simulink model "GIM81115_6_motor_model"  (R2024b)
settings: Solver=VariableStepAuto  StartTime=0.0  StopTime=10.0  RelTol=1e-3
libraries: aru_toolbox x1
settings Model: Creator=claro  LastModifiedBy=claro

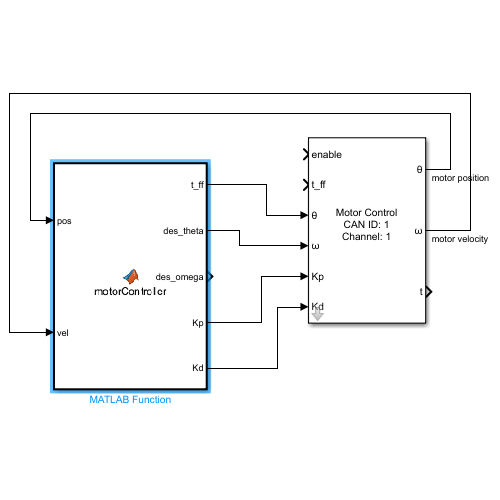
[thumbnail: Simulink's stored preview of the top-level diagram]
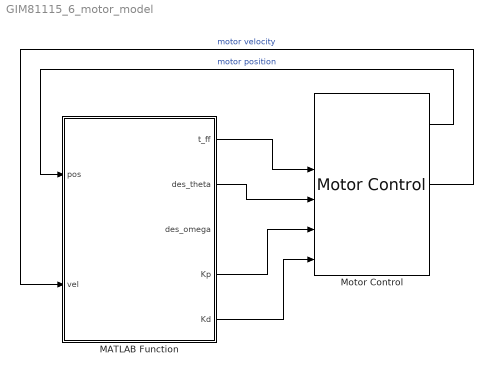
== system GIM81115_6_motor_model ==
  MATLAB Function : MATLAB Function  TreatAsAtomicUnit=on
  Motor Control : aru_toolbox/Motor Control  id=1  channel=1  offset=0
      settings: SourceProductName=ARU Toolbox
  wires:
  Motor Control/2 -> MATLAB Function/2(vel)  "motor velocity"
  Motor Control/1 -> MATLAB Function/1(pos)  "motor position"
  MATLAB Function/4(Kp) -> Motor Control/5
  MATLAB Function/5(Kd) -> Motor Control/6
  MATLAB Function/2(des_theta) -> Motor Control/4
  MATLAB Function/1(t_ff) -> Motor Control/3

== matlab function GIM81115_6_motor_model/MATLAB Function ==
  data: t_ff output; des_theta output; des_omega output; pos input; vel input; Kp output; Kd output
function [t_ff, des_theta, des_omega, Kp, Kd] = motorController(pos, vel)

    % Params
    J =  0.000072; % [kg*m^2]
    Kt = 1.84; % Torque Constant [Nm/A]
    I_max = 4.8; % Max Current [A]
    T_s = 0.1; % Settling time [s]
    zeta = 0.7; % Damping Ratio -> Underdamped
    t_limit = 0.2; % Torque Limit
    
    % Calculate Maximum Torque
    T_max = Kt * I_max;
    
    % Calcualte natural frequency
    wn = 4 / (zeta * T_s);
    
    if (pos <  -90 *pi/180) % Apply electrical break if close to mechanical limits
        des_theta = -85*pi/180;
        des_omega = 0;
        stop_distance = 5*pi/180;
        Kp = T_max/stop_distance;
        Kd = 2 * sqrt(J * Kp);
        t_ff = 0;
    elseif (pos > 90*pi/180)
        des_theta = 85*pi/180;
        des_omega = 0;
        stop_distance = 5*pi/180;
        Kp = T_max/stop_distance;
        Kd = 2 * sqrt(J * Kp);
        t_ff = 0;
    else
        des_theta = 0;
        des_omega = 0;
        Kp = J * wn^2;
        Kd = 2 * zeta * sqrt(J * Kp);
        t_ff = 0;
    end

    % Calculate comanded toruqe
    t_cmd = Kp* (des_theta - pos) + Kd * (des_omega - vel);
    t_tot = t_cmd + t_ff;

    % Scale gains 
    if abs(t_tot) > t_limit
        scale_factor = abs (t_limit/ t_tot);
        Kp = Kp * scale_factor;
        Kd = Kd * scale_factor;
    end

end
